simulink model "Ammonia_Model"  (R2023a)
settings: Solver=FixedStepAuto  StartTime=0.0  StopTime=Z  FixedStep=1/24  RelTol=1e-3
values from neighbouring files (symbols this model uses):
  c_eh = 0.85    [Model_Parameters.m]
  cc_AH2_l = 0.6    [Model_Parameters.m]
  cc_AH2_r = 0.75    [Model_Parameters.m]
  cc_AH2_z = 0.65    [Model_Parameters.m]
  cc_e = -0.85    [Model_Parameters.m]
  id_l_A = id_l*id_frac_A    (= 0.0480384)    [Model_Parameters.m]
  id_r_A = id_r*id_frac_A    (= 0.1479168)    [Model_Parameters.m]
  id_z_A = id_z*id_frac_A    (= 0.114048)    [Model_Parameters.m]
  R_ammonia = 0.025    [Model_Parameters.m]
  R_H2 = 0.05    [Model_Parameters.m]
  R_lh = 0.025    [Model_Parameters.m]
  R_ng = 0.025    [Model_Parameters.m]
  S_a_l = 0.3    [Model_Parameters.m]
  S_a_r = 0.2    [Model_Parameters.m]
  S_a_z = 0.25    [Model_Parameters.m]
libraries: fl_lib x72, nesl_utility x50, ee_lib x27
(part 2 of 2)

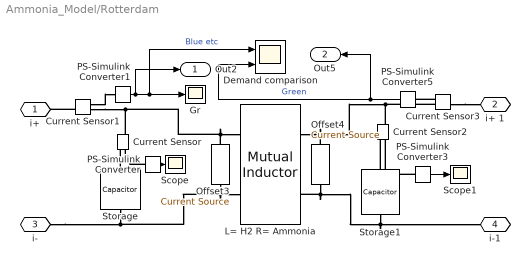
== system Ammonia_Model/Rotterdam ==
  Current Sensor{,1..3} (4 alike) : fl_lib/Electrical/Electrical Sensors/Current Sensor
  Demand comparison : Scope  NumInputPorts=2
  Gr : Scope
  L= H2 R= Ammonia : ee_lib/Passive/Transformers/Mutual Inductor  L1=L_H2_r H  L2=L_A_r H  k=cc_AH2_r  L_tol=0  enable_L1_tol=ee.enum.toleranceApplication.none  L1_tol_distribution=ee.enum.toleranceDistribution.uniform  L1_nSigma=4  enable_L2_tol=ee.enum.toleranceApplication.none  L2_tol_distribution=ee.enum.toleranceDistribution.uniform  L2_nSigma=4  r=[.001, .001] Ohm  g=[1e-09, 1e-09] 1/Ohm  enable_operating_limits=ee.enum.enable.no  operating_limit_action=ee.enum.passive.reportOpLim.warn  max_working_current=1 A  power_rating=1 W  enable_faults=ee.enum.enable.no  fault_action=simscape.enum.assert.action.none  fault_winding=ee.enum.passive.transformers.faultedWinding.primary  lambdaPercent=50  turnsShort=ee.enum.faults.faultTurnsShort.no  openCct=ee.enum.faults.faultTurnsOpenCkt.no  groundShort=ee.enum.faults.faultTurnsGroundShort.no  groundShortG=0 1/Ohm  tau_fault=1e-3 s  fault_trigger=ee.enum.faults.faultTrigger.temporal  t_fault=1 s  max_permissible_voltage=100 V  n_fail_on_voltage=1  max_permissible_current=1 A  t_fail_on_current=1 s  iL1_specify=off  iL1_priority=High  iL1=0 A  iL1_nominal_specify=off  iL1_nominal_unit=A  iL1_nominal_value=1  iL2_specify=off  iL2_priority=High  iL2=0 A  iL2_nominal_specify=off  iL2_nominal_unit=A  iL2_nominal_value=1  faulted_specify=off  faulted_priority=None  faulted=0
      settings: InternalSimscapePortConfiguration="{\"Bottom\":[],\"Left\":[{\"id\":\"p1\",\"label\":\"1+\",\"type\":\"foundation.electrical.electrical\"},{\"id\":\"n1\",\"label\":\"1-\",\"type\":\"foundation.electrical.electrical\"}],\"Right\":[{\"id\":\"p2\",\"label\":\"2+\",\"type\":\"foundation.electrical.electrical\"},{\"id\":\"n2\",\"label\":\"2-\",\"type\":\"foundation.electrical.electrical\"}],\"Top\":[]}"
  Offset3 : ee_lib/Sources/Current Source  dc_current=id_r_A*(1-S_a_r) A  ac_current=0 A  ac_shift=0 rad  ac_frequency=0 Hz  noise_mode=0  PSD=0 A^2/Hz  sample_time=1e-3 s  repeatability=1  user_seed=0  auto_seed=2984266212  i_specify=off  i_priority=None  i=0 A  i_nominal_specify=off  i_nominal_unit=A  i_nominal_value=1  v_specify=off  v_priority=None  v=0 V  v_nominal_specify=off  v_nominal_unit=V  v_nominal_value=1
  Offset4 : ee_lib/Sources/Current Source  dc_current=id_r_A*S_a_r A  ac_current=0 A  ac_shift=0 rad  ac_frequency=0 Hz  noise_mode=0  PSD=0 A^2/Hz  sample_time=1e-3 s  repeatability=1  user_seed=0  auto_seed=1361931897  i_specify=off  i_priority=None  i=0 A  i_nominal_specify=off  i_nominal_unit=A  i_nominal_value=1  v_specify=off  v_priority=None  v=0 V  v_nominal_specify=off  v_nominal_unit=V  v_nominal_value=1
  PS-Simulink Converter{,1,3,5} (4 alike) : nesl_utility/PS-Simulink Converter  PhysicalDomain=network_engine_domain  SubClassName=ps_output  LeftPortType=input  RightPortType=output  PseudoPeriodic=off  Frequencies=[]  VectorFormat=inherit  Unit=inherit  AffineConversion=off
  Scope : Scope
  Scope1 : Scope
  Storage : fl_lib/Electrical/Electrical Elements/Capacitor  c=C_g F  r=0 Ohm  g=0 1/Ohm  i_specify=off  i_priority=None  i=0 A  i_nominal_specify=off  i_nominal_unit=A  i_nominal_value=1  v_specify=off  v_priority=None  v=0 V  v_nominal_specify=off  v_nominal_unit=V  v_nominal_value=1  vc_specify=off  vc_priority=High  vc=0 V  vc_nominal_specify=off  vc_nominal_unit=V  vc_nominal_value=1
  Storage1 : fl_lib/Electrical/Electrical Elements/Capacitor  c=C_g F  r=0 Ohm  g=0 1/Ohm  i_specify=off  i_priority=None  i=0 A  i_nominal_specify=off  i_nominal_unit=A  i_nominal_value=1  v_specify=off  v_priority=None  v=0 V  v_nominal_specify=off  v_nominal_unit=V  v_nominal_value=1  vc_specify=off  vc_priority=High  vc=0 V  vc_nominal_specify=off  vc_nominal_unit=V  vc_nominal_value=1
  "i+ " : PMIOPort  Tag=PMCPort  Side=Left
  i+ 1 : PMIOPort  Tag=PMCPort  Port=2  Side=Left
  i- : PMIOPort  Tag=PMCPort  Port=3  Side=Left
  i-1 : PMIOPort  Tag=PMCPort  Port=4  Side=Left
  Out2 : Outport
  Out5 : Outport  Port=2
  wires:
  PS-Simulink Converter5/1 -> Demand comparison/2, Out5/1  "Green"
  PS-Simulink Converter/1 -> Scope/1
  PS-Simulink Converter1/1 -> Out2/1, Demand comparison/1, Gr/1  "Blue etc"
  PS-Simulink Converter3/1 -> Scope1/1
  connections:
  L= H2 R= Ammonia/RConn1 -- Offset4/LConn1 -- Storage1/LConn1 -- i-1/RConn1
  Current Sensor/LConn1 -- L= H2 R= Ammonia/LConn2 -- Offset3/RConn1 -- Current Sensor1/RConn2
  Current Sensor2/LConn1 -- L= H2 R= Ammonia/RConn2 -- Offset4/RConn1 -- Current Sensor3/RConn2
  L= H2 R= Ammonia/LConn1 -- Storage/LConn1 -- i-/RConn1 -- Offset3/LConn1
  Storage/RConn1 -- Current Sensor/RConn2
  Storage1/RConn1 -- Current Sensor2/RConn2
  PS-Simulink Converter/LConn1 -- Current Sensor/RConn1
  Current Sensor3/RConn1 -- PS-Simulink Converter5/LConn1
  Current Sensor1/LConn1 -- "i+ "/RConn1
  Current Sensor3/LConn1 -- i+ 1/RConn1
  Current Sensor1/RConn1 -- PS-Simulink Converter1/LConn1
  PS-Simulink Converter3/LConn1 -- Current Sensor2/RConn1

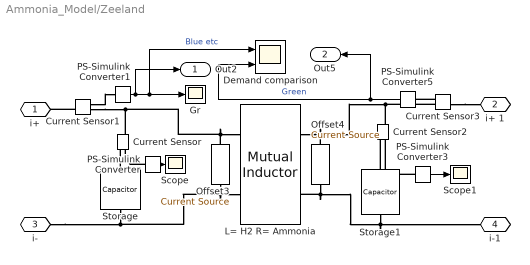
== system Ammonia_Model/Zeeland ==
  Current Sensor{,1..3} (4 alike) : fl_lib/Electrical/Electrical Sensors/Current Sensor
  Demand comparison : Scope  NumInputPorts=2
  Gr : Scope
  L= H2 R= Ammonia : ee_lib/Passive/Transformers/Mutual Inductor  L1=L_H2_z H  L2=L_A_z H  k=cc_AH2_z  L_tol=0  enable_L1_tol=ee.enum.toleranceApplication.none  L1_tol_distribution=ee.enum.toleranceDistribution.uniform  L1_nSigma=4  enable_L2_tol=ee.enum.toleranceApplication.none  L2_tol_distribution=ee.enum.toleranceDistribution.uniform  L2_nSigma=4  r=[.001, .001] Ohm  g=[1e-09, 1e-09] 1/Ohm  enable_operating_limits=ee.enum.enable.no  operating_limit_action=ee.enum.passive.reportOpLim.warn  max_working_current=1 A  power_rating=1 W  enable_faults=ee.enum.enable.no  fault_action=simscape.enum.assert.action.none  fault_winding=ee.enum.passive.transformers.faultedWinding.primary  lambdaPercent=50  turnsShort=ee.enum.faults.faultTurnsShort.no  openCct=ee.enum.faults.faultTurnsOpenCkt.no  groundShort=ee.enum.faults.faultTurnsGroundShort.no  groundShortG=0 1/Ohm  tau_fault=1e-3 s  fault_trigger=ee.enum.faults.faultTrigger.temporal  t_fault=1 s  max_permissible_voltage=100 V  n_fail_on_voltage=1  max_permissible_current=1 A  t_fail_on_current=1 s  iL1_specify=off  iL1_priority=High  iL1=0 A  iL1_nominal_specify=off  iL1_nominal_unit=A  iL1_nominal_value=1  iL2_specify=off  iL2_priority=High  iL2=0 A  iL2_nominal_specify=off  iL2_nominal_unit=A  iL2_nominal_value=1  faulted_specify=off  faulted_priority=None  faulted=0
      settings: InternalSimscapePortConfiguration="{\"Bottom\":[],\"Left\":[{\"id\":\"p1\",\"label\":\"1+\",\"type\":\"foundation.electrical.electrical\"},{\"id\":\"n1\",\"label\":\"1-\",\"type\":\"foundation.electrical.electrical\"}],\"Right\":[{\"id\":\"p2\",\"label\":\"2+\",\"type\":\"foundation.electrical.electrical\"},{\"id\":\"n2\",\"label\":\"2-\",\"type\":\"foundation.electrical.electrical\"}],\"Top\":[]}"
  Offset3 : ee_lib/Sources/Current Source  dc_current=id_z_A*(1-S_a_z) A  ac_current=0 A  ac_shift=0 rad  ac_frequency=0 Hz  noise_mode=0  PSD=0 A^2/Hz  sample_time=1e-3 s  repeatability=1  user_seed=0  auto_seed=1884392676  i_specify=off  i_priority=None  i=0 A  i_nominal_specify=off  i_nominal_unit=A  i_nominal_value=1  v_specify=off  v_priority=None  v=0 V  v_nominal_specify=off  v_nominal_unit=V  v_nominal_value=1
  Offset4 : ee_lib/Sources/Current Source  dc_current=id_z_A*S_a_z A  ac_current=0 A  ac_shift=0 rad  ac_frequency=0 Hz  noise_mode=0  PSD=0 A^2/Hz  sample_time=1e-3 s  repeatability=1  user_seed=0  auto_seed=1638781095  i_specify=off  i_priority=None  i=0 A  i_nominal_specify=off  i_nominal_unit=A  i_nominal_value=1  v_specify=off  v_priority=None  v=0 V  v_nominal_specify=off  v_nominal_unit=V  v_nominal_value=1
  PS-Simulink Converter{,1,3,5} (4 alike) : nesl_utility/PS-Simulink Converter  PhysicalDomain=network_engine_domain  SubClassName=ps_output  LeftPortType=input  RightPortType=output  PseudoPeriodic=off  Frequencies=[]  VectorFormat=inherit  Unit=inherit  AffineConversion=off
  Scope : Scope
  Scope1 : Scope
  Storage : fl_lib/Electrical/Electrical Elements/Capacitor  c=C_g F  r=0 Ohm  g=0 1/Ohm  i_specify=off  i_priority=None  i=0 A  i_nominal_specify=off  i_nominal_unit=A  i_nominal_value=1  v_specify=off  v_priority=None  v=0 V  v_nominal_specify=off  v_nominal_unit=V  v_nominal_value=1  vc_specify=off  vc_priority=High  vc=0 V  vc_nominal_specify=off  vc_nominal_unit=V  vc_nominal_value=1
  Storage1 : fl_lib/Electrical/Electrical Elements/Capacitor  c=C_g F  r=0 Ohm  g=0 1/Ohm  i_specify=off  i_priority=None  i=0 A  i_nominal_specify=off  i_nominal_unit=A  i_nominal_value=1  v_specify=off  v_priority=None  v=0 V  v_nominal_specify=off  v_nominal_unit=V  v_nominal_value=1  vc_specify=off  vc_priority=High  vc=0 V  vc_nominal_specify=off  vc_nominal_unit=V  vc_nominal_value=1
  "i+ " : PMIOPort  Tag=PMCPort  Side=Left
  i+ 1 : PMIOPort  Tag=PMCPort  Port=2  Side=Left
  i- : PMIOPort  Tag=PMCPort  Port=3  Side=Left
  i-1 : PMIOPort  Tag=PMCPort  Port=4  Side=Left
  Out2 : Outport
  Out5 : Outport  Port=2
  wires:
  PS-Simulink Converter1/1 -> Out2/1, Demand comparison/1, Gr/1  "Blue etc"
  PS-Simulink Converter5/1 -> Demand comparison/2, Out5/1  "Green"
  PS-Simulink Converter3/1 -> Scope1/1
  PS-Simulink Converter/1 -> Scope/1
  connections:
  Current Sensor/LConn1 -- Current Sensor1/RConn2 -- L= H2 R= Ammonia/LConn2 -- Offset3/RConn1
  L= H2 R= Ammonia/LConn1 -- Offset3/LConn1 -- Storage/LConn1 -- i-/RConn1
  Current Sensor2/LConn1 -- Current Sensor3/RConn2 -- L= H2 R= Ammonia/RConn2 -- Offset4/RConn1
  L= H2 R= Ammonia/RConn1 -- Offset4/LConn1 -- Storage1/LConn1 -- i-1/RConn1
  Current Sensor3/RConn1 -- PS-Simulink Converter5/LConn1
  Storage/RConn1 -- Current Sensor/RConn2
  Current Sensor1/LConn1 -- "i+ "/RConn1
  Storage1/RConn1 -- Current Sensor2/RConn2
  Current Sensor1/RConn1 -- PS-Simulink Converter1/LConn1
  PS-Simulink Converter/LConn1 -- Current Sensor/RConn1
  PS-Simulink Converter3/LConn1 -- Current Sensor2/RConn1
  Current Sensor3/LConn1 -- i+ 1/RConn1

== matlab function Ammonia_Model/MATLAB Function2 ==
  data: X input; y output
function y = fcn(X)

% % y = 0.03*sin(0.3*X)*sign(sin(X))+0.03;
% 
T=3;

w=2*pi/T;
y = 0.3*sin(w*X);
y(y<0) = 0;


end




% T=3;
% 
% w=2*pi/T;
% y = cos(w*X);
% y(y<0) = 0;

== matlab function Ammonia_Model/LH2 Shock ==
  data: X input; y output
function y= fcn(X)

%% random steps
    if X >= 150 && X < 170
        y = -0.1;
    else
        y = 0;
    end

== matlab function Ammonia_Model/NG Shock ==
  data: X input; y output
function y= fcn(X)

%% random steps
    if X >= 150 && X < 170
        y = -0.1;
    else
        y = 0;
    end

== matlab function Ammonia_Model/Yearly distribution4 ==
  data: wind_distr input; current output
function current= fcn(wind_distr)
wind=wind_distr;

%% Wind to Electricity

       
    % Power curve
    wind_speeds = [0, 2, 4, 6, 8, 10, 12, 14, 16, 18, 20, 22, 24, 26]; % Wind speed values
    power_output = [0, 0, 0.5, 1, 3.7, 4.7, 6.3, 9.5, 9.5, 9.5, 9.5, 9.5, 0, 0]; % Corresponding power output values  in MW
    %powercurve: https://www.researchgate.net/figure/Power-curve-of-the-Vestas-V164-95-turbine-including-some-technical-data-left-side-and_fig4_351600993

    % Interpolate the power curve
    power_curve = interp1(wind_speeds, power_output, wind, 'linear', 'extrap');  % 'extrap' for extrapolation MW/turbine = MW/9.5MW
    
    % Limit power output to positive values
    power_curve(power_curve < 0) = 0;

    % Apply the power curve to wind speed samples
    electricity_production = power_curve .* wind; %MW

    % Consider turbine availability and capacity if applicable
    availability_factor = 1; % Availability factor
    offshore_wind_capacity = 12e3; % Offshore wind capacity in MW (=10GW)
    nr_turbines=offshore_wind_capacity/9.5;
    % offshore_wind_capacity = 30; % Offshore wind capacity in MW

    % Produced electricity
    electricity_production_MW = electricity_production * availability_factor * nr_turbines; %MWh
    electricity_production_GW = electricity_production_MW*1e-3;

    %% Scaling to integrate within the model 
    % current = 2e7 * electricity_production;
    current = electricity_production_GW/26^2; %GWh/h

    % \ 0.0002*30/10*0.5
end
